simulink subsystem "AC_gauge_R2024a_Copy"  (R2024b)
settings: Solver=VariableStepAuto  StartTime=0.0  StopTime=10.0  RelTol=1e-3
undefined symbols (not defined in the file or in its folder): AC_tank_volume, LH2_density_table, short_pressure_vector, short_temp_vector
settings Model: Creator=MW  LastModifiedBy=MW

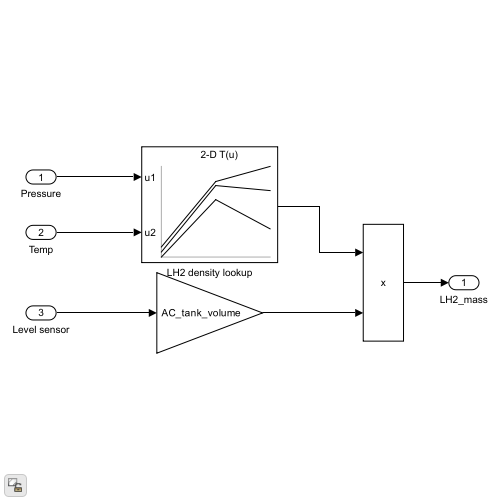
[thumbnail: Simulink's stored preview of the top-level diagram]
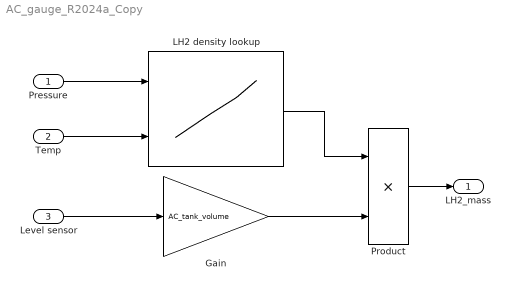
== system AC_gauge_R2024a_Copy ==
  Pressure : Inport
  Temp : Inport  Port=2
  Level sensor : Inport  Port=3
  Gain : Gain  Gain=AC_tank_volume
  LH2 density lookup : Lookup_n-D  BreakpointsForDimension1=short_pressure_vector  BreakpointsForDimension2=short_temp_vector  BeginIndexSearchUsingPreviousIndexResult=on  Table=LH2_density_table  ExtrapMethod=Clip  ApplyAccurateEfficientRounding=on  InternalRulePriority=Speed  RndMeth=Simplest
      settings: InputPortMap=u0,u1
  Product : Product
  LH2_mass : Outport
  wires:
  Pressure/1 -> LH2 density lookup/1
  Temp/1 -> LH2 density lookup/2
  LH2 density lookup/1 -> Product/1
  Level sensor/1 -> Gain/1
  Gain/1 -> Product/2
  Product/1 -> LH2_mass/1
